simulink subsystem "PvtSubSys_LATC"  (R2020b)
settings: Solver=VariableStepAuto  StartTime=0.0  StopTime=10.0  RelTol=1e-3
undefined symbols (not defined in the file or in its folder): P_Global_CharSpd_ms, P_Global_SteeringAngleRatio, P_Global_WheelBase_m, P_LCS_DetNoOverRide_DrvTrq_TH, P_LCS_DetOverRide_DrvTrq_TH, P_LCS_ESS_AngleSlope_Limit, P_LCS_ESS_LogicTest_Enable, P_LCS_ESS_NotActiveFlgDelayTime, P_LCS_ESS_NotActiveFlgDelayTimeSW, P_LCS_ESS_SteerAngleErr, P_LCS_ESS_SteerAngleFilterTime, P_LCS_ESS_TarAngleFilterTime, P_LCS_ESSAngleSW, P_LCS_ESSOverrideTime1, P_LCS_ESSOverrideTime2, P_LCS_ESSOverrideTime3, P_LCS_ESSOverrideValue1, P_LCS_ESSOverrideValue2, P_LCS_IN_Offset_Test_SW, P_LCS_IN_Offset_Test_Value, P_LCS_LATC_AngleFilterTime_s, P_LCS_LATC_CurOffsetCurve_TabX_m, P_LCS_LATC_CurOffsetCurveFliterTime_Tab_s, P_LCS_LATC_CurOffsetVehicleSpdLimitValue_degs, P_LCS_LATC_DeltaEps_Tab_s, P_LCS_LATC_DxOffset_Sw, P_LCS_LATC_ELKAngleSlope_ratio, P_LCS_LATC_ELKMaxLatAcc_ms2, P_LCS_LATC_ESSA0Dis_TabX_m, P_LCS_LATC_ESSAddAngleSlope_Tab_degs, P_LCS_LATC_ESSAESAngleSlope_Tab_degs, P_LCS_LATC_ESSAngleSlope_ratio, P_LCS_LATC_ESSMaxLatAcc_ms2, P_LCS_LATC_LCAngleSlope_ratio, P_LCS_LATC_LCAngleSlope_Tab_degs, P_LCS_LATC_LCCancleMaxLatAcc_ms2, P_LCS_LATC_LCEcoAngleSlope_ratio, P_LCS_LATC_LCEcoAngleSlope_Tab_degs, P_LCS_LATC_LCEcoMaxLatAcc_ms2, P_LCS_LATC_LCKAngleSlope_ratio, P_LCS_LATC_LCKAngleSlope_Tab_degs, P_LCS_LATC_LCKIEAngleSlope_ratio, P_LCS_LATC_LCKIEAngleSlope_Tab_degs, P_LCS_LATC_LCKIEMaxLatAcc_ms2, P_LCS_LATC_LCKMaxLatAcc_ms2, P_LCS_LATC_LCNormalAngleSlope_ratio, P_LCS_LATC_LCNormalAngleSlope_Tab_degs, P_LCS_LATC_LCNormalMaxLatAcc_ms2, P_LCS_LATC_LCSportAngleSlope_ratio, P_LCS_LATC_LCSportAngleSlope_Tab_degs, P_LCS_LATC_LCSportMaxLatAcc_ms2, P_LCS_LATC_LKAAngleSlope_ratio, P_LCS_LATC_LKAAngleSlope_Tab_degs, P_LCS_LATC_LKAMaxLatAcc_ms2, P_LCS_LATC_MatrixQ1_st, P_LCS_LATC_MatrixQ3_st, P_LCS_LATC_MatrixR_st, P_LCS_LATC_Preindex, P_LCS_LATC_PreWeight, P_LCS_LATC_StateActivAngleSlopeLimit_ratio ... (+64)
libraries: simulink x32
(part 5 of 5)

== matlab function PvtSubSys_LATC/Subsystem/LateralControl/LCS_Angle/Lateral_Control/MPC/TargetSteerAngleCalc/TargetSteerAngleCalc ==
  data: LineValid input boolean size=1; TarSteerAngle output single size=1; TarSteerAngleEnd output single size=1; Xn output single size=1; Yn output single size=1; Yawn output single size=1; Num output single size=1; J output single size=[31,1]; Jr1 output single size=[31,1]; Jq output single size=[31,1]; vxvRef input single size=1; SteerAngle input single size=1; Charspd input single size=1; WheelBase input single size=1; SteerRatio input single size=1; tDeltaEPS input single size=1; preDis input single size=1; TarSteerAngleSlope input single size=1; R1 input single size=1; Q input single size=1; TarSteerAngleK1 input single size=1; XX output; YY output; t_y output; ADDANGLE output; CurrentSteerAngleOffset input single; SteerAngleOffset_deg input; LCS_PlanX input; LCS_PlanY input; preindex input size=[1 7]; preWeight input size=[1 7]; dxoffset_SW input
function [TarSteerAngle,TarSteerAngleEnd,Xn,Yn,Yawn,Num,J,Jr1,Jq,XX,YY,t_y,ADDANGLE] = ...
    TargetSteerAngleCalc(LineValid,vxvRef,SteerAngle,Charspd,WheelBase,SteerRatio,tDeltaEPS,preDis,TarSteerAngleSlope,R1,Q,...
    TarSteerAngleK1,CurrentSteerAngleOffset,SteerAngleOffset_deg,...
    LCS_PlanX,LCS_PlanY,preindex,preWeight,dxoffset_SW)

StrToWhlFac = 57.3*SteerRatio;  %弧度转换角度
SteerAngleDt = single(TarSteerAngleSlope*50);  %每个周期方向盘转动变化率(°/s)
dxOffset = single(2.1);  %车辆质心位置
J = single(zeros(31,1));
Jr1 = single(zeros(31,1));
Jq = single(zeros(31,1));
Num = single(0); 
XX = single(zeros(1,20));
YY = single(zeros(1,20));
t_y = single(zeros(1,20));
ADDANGLE= 0;

deltaAngle = [-45.5, -34.4, -25.3, -18.0, -12.3, -8.0,...
    -4.9, -2.8, -1.5, -0.8, -0.5, -0.4, -0.3, -0.2, -0.1, ...
    0, 0.1, 0.2, 0.3, 0.4, 0.5, 0.8, 1.5, 2.8,...
    4.9, 8.0, 12.3, 18.0, 25.3, 34.4, 45.5];

vRef = max(vxvRef,single(0.1));

if LineValid
    % 20 Calculate Cycle
    disStep = preDis/single(49);         %将规划轨迹均分50等份
    SteerAngleMa = single(zeros(31,20)); %方向盘转角矩阵
    YawMa = single(zeros(31,20));        %车身朝向角
    YiMa = single(zeros(31,20));         %横坐标
    XiMa = single(zeros(31,20));         %纵坐标
    yValid = true(31,1);
    Jmin =single(-1);
    Num = single(0);

    for k=single(1:31)
        SteerAngleRaw = SteerAngle + deltaAngle(k);  %方向盘实际有效转角+预期方向盘增量
        tD = disStep/vRef;                           %行驶完每一份规划轨迹所用的时间（预测步长）
        %% 推算每条轨迹下每个轨迹点处方向盘转角
        SteerAngleMa(k,1) =  TarSteerAngleK1;        %计算31条轨迹起始位置的方向盘转角
        for i=2:20                                   %每条轨迹的20个轨迹点之间的预测步长选择（变步长）
            if i<=5
                tDelta = tD;
            elseif i<=10
                tDelta = 2*tD;
            elseif i<=15
                tDelta = 3*tD;
            else
                tDelta = 4*tD;
            end
            if SteerAngleRaw>SteerAngle    %判断转向方向  方向盘转角左正右负  
                SteerAngleMa(k,i) = SteerAngleMa(k,1) + tDelta*single((i-1))*SteerAngleDt;%计算每条轨迹下的20个方向盘转角
                SteerAngleMa(k,i) = min(SteerAngleMa(k,i),SteerAngleRaw);% 
            else
                SteerAngleMa(k,i) = SteerAngleMa(k,1) - tDelta*(single(i-1))*SteerAngleDt;
                SteerAngleMa(k,i) = max(SteerAngleMa(k,i),SteerAngleRaw);
            end
        end
        %% 计算每条轨迹下起始点的坐标及车身朝向角
        if vRef<1
            YawMa(k,1) = tDeltaEPS*vRef*tan(0.5*(SteerAngle + TarSteerAngleK1)/StrToWhlFac)/WheelBase; % 计算每一条推算轨迹起始位置的车身朝向角（单位：rad）
        else
            AckConst = min((single(1)+vRef*vRef/(Charspd*Charspd))*WheelBase/max(single(1),vRef),single(32767));          %计算稳态横摆角速度增益 （单位：s）
            YawMa(k,1) = 0.5*tDeltaEPS*(SteerAngle + TarSteerAngleK1)/(AckConst*StrToWhlFac);     % 计算每一条推算轨迹起始位置的车身朝向角(角度)
        end
        XiMa(k,1) = tDeltaEPS*vRef*cos(YawMa(k,1));%推算第一步纵向坐标
        YiMa(k,1) = tDeltaEPS*vRef*sin(YawMa(k,1));%推算第一步横向坐标
        %% 
        uDelta = SteerAngleRaw - SteerAngle;

        % t_Start =single(18);
        t_End = single(19); 
        for i=1:t_End
            if i<=5
                disStepFac = single(1);
            elseif i<=10
                disStepFac = single(2);
            elseif i<=15
                disStepFac = single(3);
            else
                disStepFac = single(4);
            end
            if vRef<1
                t_kap = tan(SteerAngleMa(k,i)/StrToWhlFac)/WheelBase;  %计算每一个方向盘转角下对应的曲率
                YawMa(k,i+1) = YawMa(k,i) + disStepFac*disStep*t_kap;  %计算每一条推算轨迹除起始位置的车身朝向角
            else
                tStep = disStepFac*disStep/vRef;
                AckConst = min((single(1)+vRef*vRef/(Charspd*Charspd))*WheelBase/vRef,single(32767));
                YawRate = SteerAngleMa(k,i)/(AckConst*StrToWhlFac); %前轮转角变化率
                YawMa(k,i+1) = YawMa(k,i) + YawRate*tStep;     %计算每一条推算轨迹除起始位置的前轮转角
            end
            
            if (YawMa(k,i+1)>single(1.2))||(YawMa(k,i+1)<single(-1.2)) %筛选推算轨迹
                yValid(k) = false;
            else
                XiMa(k,i+1) = XiMa(k,i) + disStepFac*disStep *cos(0.5*(YawMa(k,i)+YawMa(k,i+1))); %计算每一个推算点的纵向坐标
                YiMa(k,i+1) = YiMa(k,i) + disStepFac*disStep *sin(0.5*(YawMa(k,i)+YawMa(k,i+1))); %计算每一个推算点的横向坐标
            end
        end
        
        if yValid(k) == true
            % 推算车辆中心点的位置坐标
            if dxoffset_SW == 1
                for i = single(1):single(1):single(20)
                    XiMa(k,i) = XiMa(k,i) + dxOffset*cos(YawMa(k,i));
                    YiMa(k,i) = YiMa(k,i) + dxOffset*sin(YawMa(k,i));
                end
            end
            % 计算损失量
            preXi = XiMa(k,preindex);
            preYi = YiMa(k,preindex);
            PlanYi = interp1(LCS_PlanX',LCS_PlanY',preXi,'linear');
            Jr1(k) = R1*sum(((preYi - PlanYi).^2).*preWeight);      %规划点与控制点之间的横向误差最小（说明两个轨迹贴合程度较高）
            J(k) = J(k) + Jr1(k);
        end
        
        %% 第K步的损失量
        Jq(k) = Q*uDelta^2;
        J(k) = J(k) + Jq(k);
        
        if (yValid(k)==true)
            if Jmin<0
                Jmin = J(k);
                Num = k;
            else
                if k<=16
                    if J(k)<=Jmin
                        Jmin = J(k);
                        Num = k;
                    end
                else
                    if J(k)<Jmin
                        Jmin = J(k);
                        Num = k;
                    end
                end
            end
        end
        
    end
    
    TarSteerAngleEnd = SteerAngle + deltaAngle(Num); 
    TarSteerAngle = min(TarSteerAngleK1 + TarSteerAngleSlope,max(TarSteerAngleK1 - TarSteerAngleSlope,TarSteerAngleEnd));
   
    Xn = XiMa(Num,t_End);
    Yn = YiMa(Num,t_End);
    Yawn = YawMa(Num,t_End);
    XX =  XiMa(Num,:);
    YY =  YiMa(Num,:);
    
    ADDANGLE=deltaAngle(Num);
else
    TarSteerAngle = SteerAngle+SteerAngleOffset_deg-CurrentSteerAngleOffset;
    TarSteerAngleEnd = SteerAngle;
    Xn = single(0);
    Yn = single(0);
    Yawn = single(0);
end
end

== matlab function PvtSubSys_LATC/Subsystem/LateralControl/LCS_Angle/Lateral_Control/Dynamic_Model_LQR/SteerAngSlopeCalc/MATLAB Function3 ==
  data: delytime input uint16; TarDangerLevel input uint8; TarDangerLevelK1 input uint8; FLg output uint8; FLgK1 input uint8; CntK1 input uint16; Cnt output uint16
function [FLg,Cnt] = AngSlopeCalc(delytime,TarDangerLevel,TarDangerLevelK1,FLgK1,CntK1)

Cnt = min(CntK1 + uint16(1),delytime);
if Cnt== delytime
    FLg = uint8(0);
else
    FLg = FLgK1;
end
%FLg = FLgK1;
%% 
if TarDangerLevel==uint8(1) && TarDangerLevelK1==0  % NO function 2 LCK (TarDangerLevelK1==0)
    Cnt =uint16(0);
    FLg = uint8(1);
end

if  TarDangerLevel==uint8(3) && (TarDangerLevelK1==uint8(1)||TarDangerLevelK1==uint8(2)) % LCK/IE 2 LC_Normal
    Cnt =uint16(0);
    FLg = uint8(2);
end

if  TarDangerLevel==uint8(7) && (TarDangerLevelK1==uint8(1)||TarDangerLevelK1==uint8(2)) % LCK/IE 2 LC_Eco
    Cnt =uint16(0);
    FLg = uint8(3);
end

if  TarDangerLevel==uint8(8) && (TarDangerLevelK1==uint8(1)||TarDangerLevelK1==uint8(2)) % LCK/IE 2 LC_sport
    Cnt =uint16(0);
    FLg = uint8(4);
end
if  TarDangerLevel==uint8(6) && (TarDangerLevelK1==uint8(1)||TarDangerLevelK1==uint8(2)) % LCK/IE 2 ESS 后期添加配和ESS Slope 一起调试
    Cnt =uint16(0);
    FLg = uint8(5);
end

== matlab function PvtSubSys_LATC/Subsystem/LateralControl/LCS_Angle/Lateral_Control/Dynamic_Model_LQR/Understeer_Offset_Calc/YOD_Ackman ==
  data: AckConst output; VxvRef input; Vch input; WheelBase input; AlpWheelAngle input; PsiDtAckK1 input single; PsiDtAck output
function [AckConst,PsiDtAck] = Ackman(VxvRef,Vch,WheelBase,AlpWheelAngle,PsiDtAckK1)
%#codegen
if VxvRef==uint8(0)%转换常数数据类型
    PsiDtAckRaw = single(0);%转换常数数据类型
    AckConst = single(1);%转换常数数据类型
else
    AckConst = min((single(1)+VxvRef*VxvRef/(Vch*Vch))*WheelBase/VxvRef,single(32767));%转换常数数据类型
    PsiDtAckRaw = AlpWheelAngle/AckConst;
end
PsiDtAck = (single(0.02/0.1))*(PsiDtAckRaw-PsiDtAckK1)+PsiDtAckK1;%转换常数数据类型
